simulink model "TokenRing"  (R2022a)
settings: Solver=VariableStepAuto  StartTime=0.0  StopTime=700  RelTol=1e-3
undefined symbols (not defined in the file): m, n
settings Model: Creator=aurisb  LastModifiedBy=aurisb

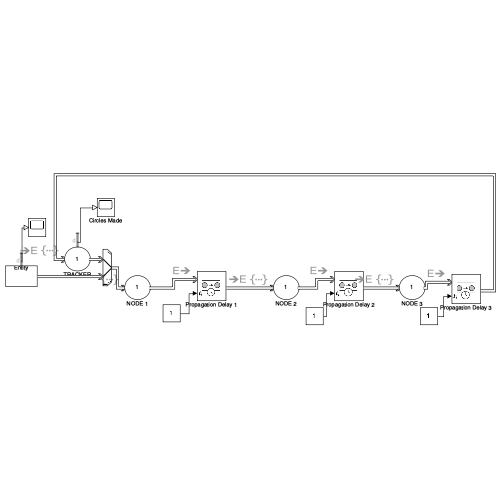
[thumbnail: Simulink's stored preview of the top-level diagram]
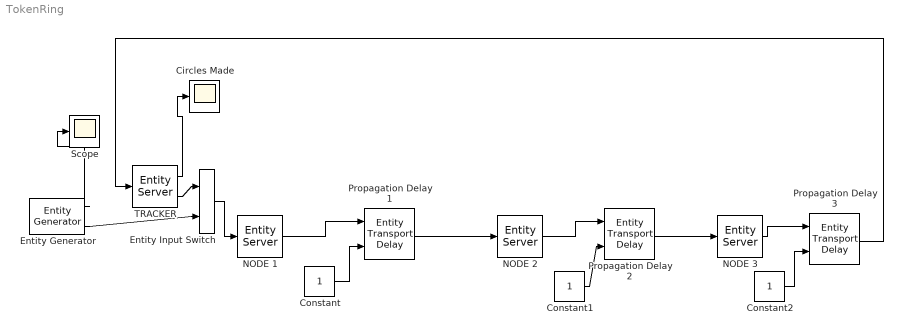
== system TokenRing ==
  Circles Made : Scope
  Constant : Constant
  Constant1 : Constant
  Constant2 : Constant
  Entity Input Switch : EntityInputSwitch  InputPortMessageModes=m,m  OutputPortMessageModes=m
  Entity Generator : EntityGenerator  OutputPortMessageModes=n,m  Period=inf  AttributeName=token|ACK|Source|Destination|ServiceTimeValue|FrameSize|data|totalPasses|usefulPasses  AttributeInitialValue=0|0|1|1|0|4472|1|1|1  NumberEntitiesDeparted=on  EntityType=Structured  EntityTypeName=Entity
      settings: OutputPortMap=o0,o3
  NODE 1 : EntityServer  InputPortMessageModes=m  OutputPortMessageModes=m  Capacity=1  ServiceTimeSource=Attribute  ServiceTimeValue=5  ServiceTimeAttributeName=ServiceTimeValue  EntryAction=|
      | myid = 1;
      | totalNodes = 3;
      | persistent dataToSend;
      | if isempty(dataToSend)
      | 	dataToSend = 58136; %17888;
      | end
      | 
      | entity.totalPasses = entity.totalPasses+1;
      | 
      | %If token is an ACK meant for you, free it 
      | if entity.ACK == 1
      | 	if entity.Destination == myid %CHANGE
      | 		entity.usefulPasses = entity.usefulPasses+1;
      | 		disp("Node " + myid + " received ACK from " + entity.Source + ". Releasing free token.");
      | 		entity.ACK=0;
      | 		entity.token=0;
      |     else
      |     	disp("Node " + myid + " passing along ACK to " + entity.Destination + ".");
      |     end
      | end
      |     
      | 
      | %If token is not free token
      | if entity.token == 1
      | 	%if it is meant for you
      | 	if entity.Destination == myid %CHANGE
      | 		entity.usefulPasses = entity.usefulPasses+1;
      | 		disp("Node " + myid + " received data, sending ACK back to " + entity.Source);
      | 
      | 		%if it is meant for you as an ACK, free it
      | 		if entity.ACK==1
      | 			entity.ACK=0;
      | 			entity.token=0;
      | 		%if it is meant for you as a message, send back an ACK
      | 		else
      | 			entity.ACK=1;
      | 			entity.Destination = entity.Source;
      | 			entity.Source=myid; %CHANGE
      | 	    end
      | 
      | 	%if it is meant for someone else, pass it on
      | 	else
      | 		disp("Node " + myid + " passing along token from " + entity.Source + " to " + entity.Destination + ".");
      | 		%do nothing and pass it on
      | 	end
      | end
      | 
      | %If it it is a free token, send data
      | if entity.token == 0 && dataToSend > 0
      | 
      | 	entity.token=1;
      | 	destinationPossibilities = setdiff(1:totalNodes, myid);
      | 	entity.Destination = destinationPossibilities(ceil(numel(destinationPossibilities) * rand));
      | 	
      | 	%entity.Destination = randi([1,totalNodes-1]);
      | 	%if entity.Destination == myid
      | 	%		entity.Destination = anotherid;
      | 	%end
      | 	entity.Source=myid; %CHANGE
      | 	dataToSend = dataToSend-4472;
      | 	entity.data=4472;
      | 	disp("Node "+myid+ " sending 4472 bytes of data to " + entity.Destination+ ". Node "+ myid + " has " + dataToSend + " bytes of data remaining to send.");
      | else if entity.token == 0
      | 	disp("Node " + myid + " has no data to send, passing token along.");
      | end
  NODE 2 : EntityServer  InputPortMessageModes=m  OutputPortMessageModes=m  Capacity=1  ServiceTimeSource=Attribute  ServiceTimeValue=5  ServiceTimeAttributeName=ServiceTimeValue  EntryAction=|
      | myid = 2;
      | totalNodes = 3;
      | persistent dataToSend;
      | if isempty(dataToSend)
      | 	dataToSend = 58136;
      | end
      | 
      | entity.totalPasses = entity.totalPasses+1;
      | 
      | %If token is an ACK meant for you, free it 
      | if entity.ACK == 1
      | 	if entity.Destination == myid %CHANGE
      | 		entity.usefulPasses = entity.usefulPasses+1;
      | 		disp("Node " + myid + " received ACK from " + entity.Source + ". Releasing free token.");
      | 		entity.ACK=0;
      | 		entity.token=0;
      |     else
      |     	disp("Node " + myid + " passing along ACK to " + entity.Destination + ".");
      |     end
      | end
      |     
      | 
      | %If token is not free token
      | if entity.token == 1
      | 	%if it is meant for you
      | 	if entity.Destination == myid %CHANGE
      | 		entity.usefulPasses = entity.usefulPasses+1;
      | 		disp("Node " + myid + " received data, sending ACK back to " + entity.Source);
      | 
      | 		%if it is meant for you as an ACK, free it
      | 		if entity.ACK==1
      | 			entity.ACK=0;
      | 			entity.token=0;
      | 		%if it is meant for you as a message, send back an ACK
      | 		else
      | 			entity.ACK=1;
      | 			entity.Destination = entity.Source;
      | 			entity.Source=myid; %CHANGE
      | 	    end
      | 
      | 	%if it is meant for someone else, pass it on
      | 	else
      | 		disp("Node " + myid + " passing along token from " + entity.Source + " to " + entity.Destination + ".");
      | 		%do nothing and pass it on
      | 	end
      | end
      | 
      | %If it it is a free token, send data
      | if entity.token == 0 && dataToSend > 0
      | 
      | 	entity.token=1;
      | 	destinationPossibilities = setdiff(1:totalNodes, myid);
      | 	entity.Destination = destinationPossibilities(ceil(numel(destinationPossibilities) * rand));
      | 	
      | 	%entity.Destination = randi([1,totalNodes-1]);
      | 	%if entity.Destination == myid
      | 	%		entity.Destination = anotherid;
      | 	%end
      | 	entity.Source=myid; %CHANGE
      | 	dataToSend = dataToSend-4472;
      | 	entity.data=4472;
      | 	disp("Node "+myid+ " sending 4472 bytes of data to " + entity.Destination+ ". Node 1 has " + dataToSend + " bytes of data remaining to send.");
      | else if entity.token == 0
      | 	disp("Node " + myid + " has no data to send, passing token along.");
      | end
  NODE 3 : EntityServer  InputPortMessageModes=m  OutputPortMessageModes=m  Capacity=1  ServiceTimeSource=Attribute  ServiceTimeValue=5  ServiceTimeAttributeName=ServiceTimeValue  EntryAction=|
      | myid = 3;
      | totalNodes = 3;
      | persistent dataToSend;
      | if isempty(dataToSend)
      | 	dataToSend = 62608;
      | end
      | 
      | entity.totalPasses = entity.totalPasses+1;
      | 
      | %If token is an ACK meant for you, free it 
      | if entity.ACK == 1
      | 	if entity.Destination == myid %CHANGE
      | 		entity.usefulPasses = entity.usefulPasses+1;
      | 		disp("Node " + myid + " received ACK from " + entity.Source + ". Releasing free token.");
      | 		entity.ACK=0;
      | 		entity.token=0;
      |     else
      |     	disp("Node " + myid + " passing along ACK to " + entity.Destination + ".");
      |     end
      | end
      |     
      | 
      | %If token is not free token
      | if entity.token == 1
      | 	%if it is meant for you
      | 	if entity.Destination == myid %CHANGE
      | 		entity.usefulPasses = entity.usefulPasses+1;
      | 		disp("Node " + myid + " received data, sending ACK back to " + entity.Source);
      | 
      | 		%if it is meant for you as an ACK, free it
      | 		if entity.ACK==1
      | 			entity.ACK=0;
      | 			entity.token=0;
      | 		%if it is meant for you as a message, send back an ACK
      | 		else
      | 			entity.ACK=1;
      | 			entity.Destination = entity.Source;
      | 			entity.Source=myid; %CHANGE
      | 	    end
      | 
      | 	%if it is meant for someone else, pass it on
      | 	else
      | 		disp("Node " + myid + " passing along token from " + entity.Source + " to " + entity.Destination + ".");
      | 		%do nothing and pass it on
      | 	end
      | end
      | 
      | %If it it is a free token, send data
      | if entity.token == 0 && dataToSend > 0
      | 
      | 	entity.token=1;
      | 	destinationPossibilities = setdiff(1:totalNodes, myid);
      | 	entity.Destination = destinationPossibilities(ceil(numel(destinationPossibilities) * rand));
      | 	
      | 	%entity.Destination = randi([1,totalNodes-1]);
      | 	%if entity.Destination == myid
      | 	%		entity.Destination = anotherid;
      | 	%end
      | 	entity.Source=myid; %CHANGE
      | 	dataToSend = dataToSend-4472;
      | 	entity.data=4472;
      | 	disp("Node "+myid+ " sending 4472 bytes of data to " + entity.Destination+ ". Node 1 has " + dataToSend + " bytes of data remaining to send.");
      | else if entity.token == 0
      | 	disp("Node " + myid + " has no data to send, passing token along.");
      | end
  Propagation Delay 1 : EntityTransportDelay  InputPortMessageModes=m,n  OutputPortMessageModes=m
  Propagation Delay 2 : EntityTransportDelay  InputPortMessageModes=m,n  OutputPortMessageModes=m
  Propagation Delay 3 : EntityTransportDelay  InputPortMessageModes=m,n  OutputPortMessageModes=m
  Scope : Scope
  TRACKER : EntityServer  InputPortMessageModes=m  OutputPortMessageModes=n,m  Capacity=1  ServiceTimeValue=0  EntryAction=|  NumberEntitiesDeparted=on
      | persistent loops;
      | if isempty(loops)
      | 	loops = 0;
      | end
      | loops = loops + 1;
      | coder.extrinsic('get_param');
      | disp(get_param('TokenRing','SimulationTime'));
      | disp("[TRACKER] Loops done around ring: " + loops + ".");
      | disp("[TRACKER] Total Passes: " + entity.totalPasses + ". Useful Passes: " + entity.usefulPasses + ".");
      settings: OutputPortMap=o0,o9
  wires:
  NODE 3/1 -> Propagation Delay 3/1
  NODE 2/1 -> Propagation Delay 2/1
  Entity Generator/2 -> Entity Input Switch/2
  Entity Input Switch/1 -> NODE 1/1
  Entity Generator/1 -> Scope/1
  TRACKER/2 -> Entity Input Switch/1
  TRACKER/1 -> Circles Made/1
  NODE 1/1 -> Propagation Delay 1/1
  Propagation Delay 1/1 -> NODE 2/1
  Propagation Delay 2/1 -> NODE 3/1
  Propagation Delay 3/1 -> TRACKER/1
  Constant/1 -> Propagation Delay 1/2
  Constant1/1 -> Propagation Delay 2/2
  Constant2/1 -> Propagation Delay 3/2
